simulink model "ControlLed"  (R2024b)
settings: Solver=VariableStepAuto  StartTime=0.0  StopTime=inf  RelTol=1e-3
libraries: arduinolib x3
settings Model: Creator=m4ttn  LastModifiedBy=m4ttn

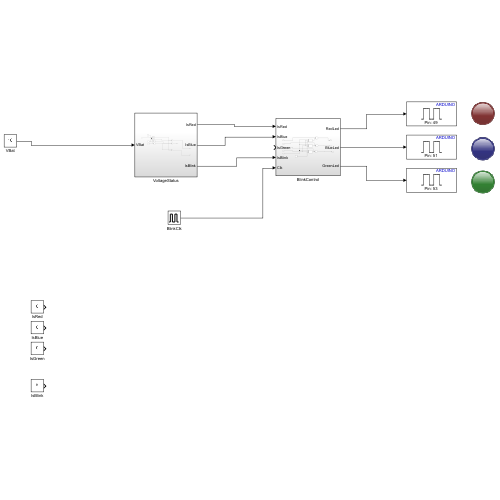
[thumbnail: Simulink's stored preview of the top-level diagram]
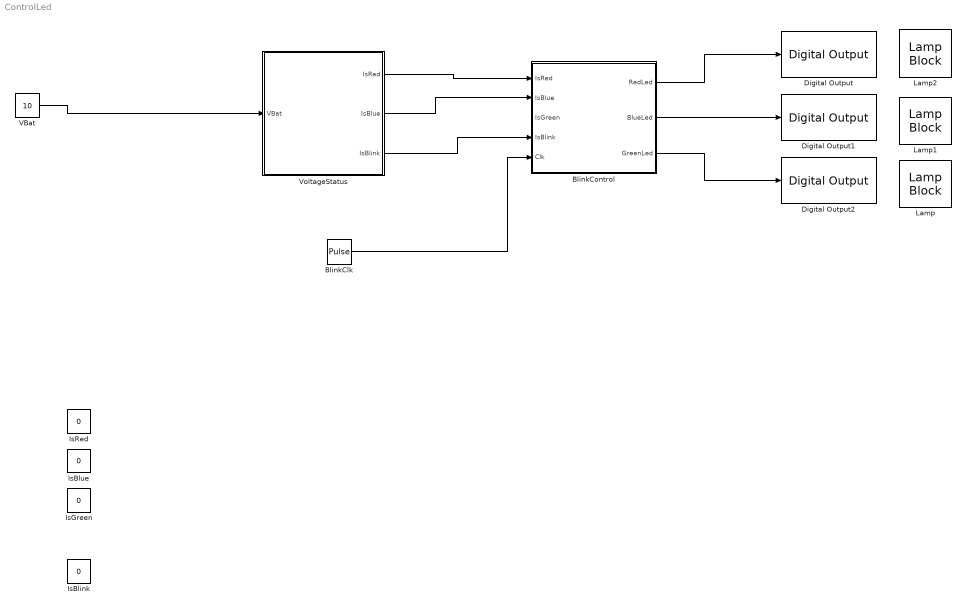
== system ControlLed ==
  BlinkClk : DiscretePulseGenerator  PulseType=Time based  Period=1  PulseWidth=50
  BlinkControl : Subsystem
  Digital Output : arduinolib/Digital Output  pinNumber=49  Direction=output  blockPlatform=arduino
  Digital Output1 : arduinolib/Digital Output  pinNumber=51  Direction=output  blockPlatform=arduino
  Digital Output2 : arduinolib/Digital Output  pinNumber=53  Direction=output  blockPlatform=arduino
  IsBlink : Constant  Value=0
  IsBlue : Constant  Value=0
  IsGreen : Constant  Value=0
  IsRed : Constant  Value=0
  Lamp : LampBlock  LabelPosition=Hide
  Lamp1 : LampBlock  LabelPosition=Hide
  Lamp2 : LampBlock  LabelPosition=Hide
  VBat : Constant  Value=10
  VoltageStatus : Subsystem
  wires:
  BlinkControl/1(RedLed) -> Digital Output/1
  BlinkControl/2(BlueLed) -> Digital Output1/1
  BlinkControl/3(GreenLed) -> Digital Output2/1
  VBat/1 -> VoltageStatus/1(VBat)
  VoltageStatus/2(IsBlue) -> BlinkControl/2(IsBlue)
  VoltageStatus/3(IsBlink) -> BlinkControl/4(IsBlink)
  VoltageStatus/1(IsRed) -> BlinkControl/1(IsRed)
  BlinkClk/1 -> BlinkControl/5(Clk)

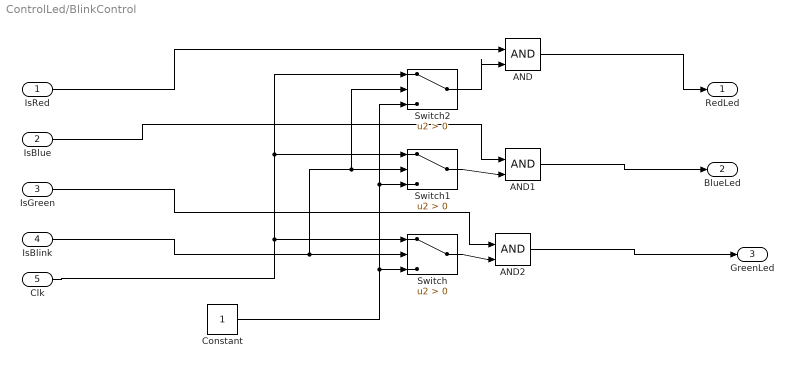
== system ControlLed/BlinkControl ==
  IsRed : Inport  OutDataTypeStr=boolean
  IsBlue : Inport  Port=2
  IsGreen : Inport  Port=3
  IsBlink : Inport  Port=4
  Clk : Inport  Port=5
  AND : Logic  IconShape=distinctive  AllPortsSameDT=off  OutDataTypeStr=boolean
  AND1 : Logic  IconShape=distinctive  AllPortsSameDT=off  OutDataTypeStr=boolean
  AND2 : Logic  IconShape=distinctive  AllPortsSameDT=off  OutDataTypeStr=boolean
  Constant : Constant  OutDataTypeStr=boolean
  Switch : Switch  Criteria=u2 > Threshold  SaturateOnIntegerOverflow=off  InputSameDT=off
  Switch1 : Switch  Criteria=u2 > Threshold  SaturateOnIntegerOverflow=off  InputSameDT=off
  Switch2 : Switch  Criteria=u2 > Threshold  SaturateOnIntegerOverflow=off  InputSameDT=off
  RedLed : Outport
  BlueLed : Outport  Port=2
  GreenLed : Outport  Port=3
  wires:
  IsBlink/1 -> Switch2/2, Switch1/2, Switch/2
  IsRed/1 -> AND/1
  AND/1 -> RedLed/1
  Switch2/1 -> AND/2
  Switch1/1 -> AND1/2
  Switch/1 -> AND2/2
  IsBlue/1 -> AND1/1
  IsGreen/1 -> AND2/1
  AND1/1 -> BlueLed/1
  AND2/1 -> GreenLed/1
  Clk/1 -> Switch/1, Switch1/1, Switch2/1
  Constant/1 -> Switch/3, Switch1/3, Switch2/3

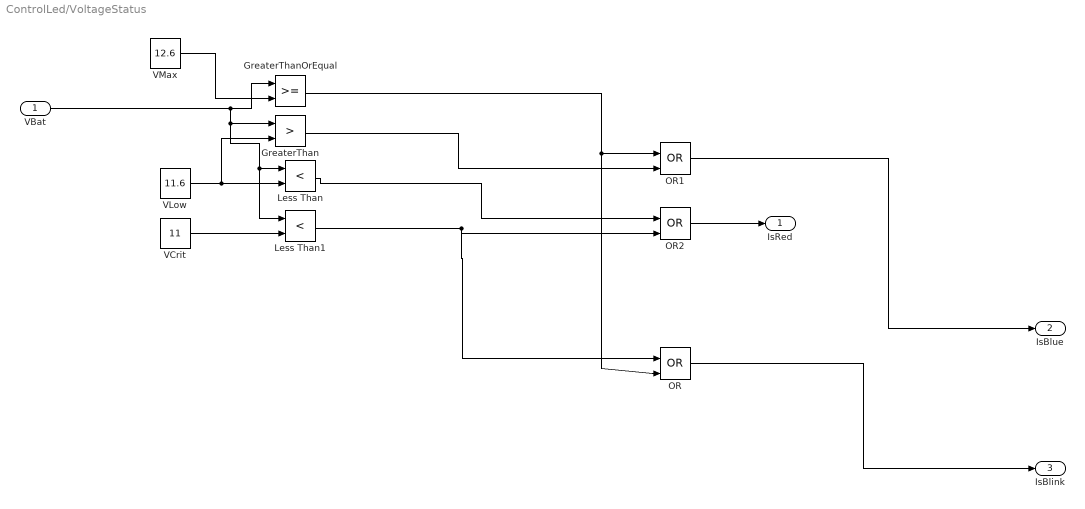
== system ControlLed/VoltageStatus ==
  VBat : Inport
  GreaterThan : RelationalOperator  Operator=>  OutDataTypeStr=boolean  RndMeth=Simplest  InputSameDT=off
  GreaterThanOrEqual : RelationalOperator  OutDataTypeStr=boolean  RndMeth=Simplest  InputSameDT=off
  Less Than : RelationalOperator  Operator=<  OutDataTypeStr=boolean  RndMeth=Simplest  InputSameDT=off
  Less Than1 : RelationalOperator  Operator=<  OutDataTypeStr=boolean  RndMeth=Simplest  InputSameDT=off
  OR : Logic  Operator=OR  IconShape=distinctive  AllPortsSameDT=off  OutDataTypeStr=boolean
  OR1 : Logic  Operator=OR  IconShape=distinctive  AllPortsSameDT=off  OutDataTypeStr=boolean
  OR2 : Logic  Operator=OR  IconShape=distinctive  AllPortsSameDT=off  OutDataTypeStr=boolean
  VCrit : Constant  Value=11
  VLow : Constant  Value=11.6
  VMax : Constant  Value=12.6
  IsRed : Outport
  IsBlue : Outport  Port=2
  IsBlink : Outport  Port=3
  wires:
  Less Than/1 -> OR2/1
  VLow/1 -> GreaterThan/2, Less Than/2
  Less Than1/1 -> OR2/2, OR/1
  VBat/1 -> GreaterThan/1, Less Than1/1, Less Than/1, GreaterThanOrEqual/1
  VMax/1 -> GreaterThanOrEqual/2
  OR2/1 -> IsRed/1
  GreaterThanOrEqual/1 -> OR1/1, OR/2
  GreaterThan/1 -> OR1/2
  VCrit/1 -> Less Than1/2
  OR/1 -> IsBlink/1
  OR1/1 -> IsBlue/1
